simulink model "ochrana_proti_rovnakym_vstupom"  (Simulink 8.7)
settings: Solver=VariableStepAuto  StartTime=0.0  StopTime=10.0  RelTol=1e-3
settings Model: Creator=Jozko Mrkvicka  LastModifiedBy=Jozko Mrkvicka
settings DataIOCC: LimitDataPoints=off  SaveFormat=Dataset
settings DebuggingCC: UnderspecifiedInitializationDetection=Simplified  MergeDetectMultiDrivingBlocksExec=error
settings HardwareCC: ProdBitPerPointer=64  ProdLargestAtomicFloat=Float  ProdIntDivRoundTo=Zero  ProdEndianess=LittleEndian  ProdWordSize=64  ProdHWDeviceType=Intel->x86-64 (Windows64)
settings ModelReferenceCC: PropagateSignalLabelsOutOfModel=on
settings ConfigComp: CovModelRefEnable=off

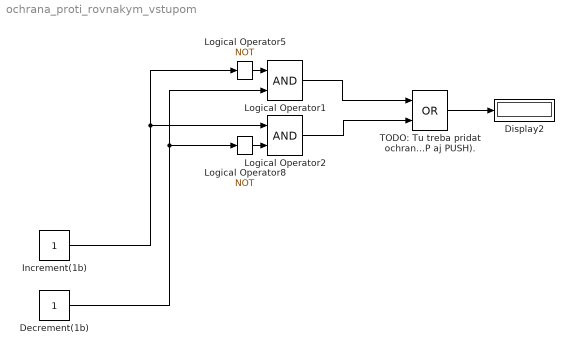
== system ochrana_proti_rovnakym_vstupom ==
  Decrement(1b) : Constant  OutDataTypeStr=boolean
  Display2 : Display
  Increment(1b) : Constant  OutDataTypeStr=boolean
  Logical Operator1 : Logic  IconShape=distinctive  AllPortsSameDT=off  OutDataTypeStr=boolean
  Logical Operator2 : Logic  IconShape=distinctive  AllPortsSameDT=off  OutDataTypeStr=boolean
  Logical Operator5 : Logic  Operator=NOT  IconShape=distinctive  AllPortsSameDT=off  OutDataTypeStr=boolean
  Logical Operator8 : Logic  Operator=NOT  IconShape=distinctive  AllPortsSameDT=off  OutDataTypeStr=boolean
  TODO: Tu treba pridat ochranu  proti stavu ked  pridu dve jednotky  (naraz instrukcia POP aj PUSH). : Logic  Operator=OR  IconShape=distinctive  AllPortsSameDT=off  OutDataTypeStr=boolean
  wires:
  Logical Operator1/1 -> TODO: Tu treba pridat ochranu  proti stavu ked  pridu dve jednotky  (naraz instrukcia POP aj PUSH)./1
  TODO: Tu treba pridat ochranu  proti stavu ked  pridu dve jednotky  (naraz instrukcia POP aj PUSH)./1 -> Display2/1
  Logical Operator2/1 -> TODO: Tu treba pridat ochranu  proti stavu ked  pridu dve jednotky  (naraz instrukcia POP aj PUSH)./2
  Logical Operator5/1 -> Logical Operator1/1
  Decrement(1b)/1 -> Logical Operator8/1, Logical Operator1/2
  Increment(1b)/1 -> Logical Operator5/1, Logical Operator2/1
  Logical Operator8/1 -> Logical Operator2/2
